simulink library "Lib_PFSys_GenericGenerator_NoSolver"  (R2019b)
settings: Solver=ode45  StartTime=0.0  StopTime=10.0  RelTol=1e-3  EnableMultiTasking=on
Description:
  | Thomas Modules
settings Model: Creator=jwchapm2  LastModifiedBy=mebell
settings DataIOCC: LimitDataPoints=on  SaveFormat=Array  ReturnWorkspaceOutputs=off
settings OptimizationCC: ExpressionDepthLimit=2147483647  LifeSpan=inf
settings DebuggingCC: UnderspecifiedInitializationDetection=Classic  MergeDetectMultiDrivingBlocksExec=none  SolverPrmCheckMsg=warning  StateNameClashWarn=warning  SFUnexpectedBacktrackingDiag=warning  SFNoUnconditionalDefaultTransitionDiag=warning  SFExecutionAtInitializationDiag=none  ArithmeticOperatorsInVariantConditions=warning
settings HardwareCC: ProdBitPerPointer=32  ProdBitPerSizeT=32  ProdBitPerPtrDiffT=32  ProdLargestAtomicFloat=None  ProdIntDivRoundTo=Undefined  ProdEndianess=Unspecified  ProdWordSize=32  ProdHWDeviceType=32-bit Generic
settings ModelReferenceCC: PropagateSignalLabelsOutOfModel=off
settings SFSimCC: SimUseLocalCustomCode=off  CustomCodeUndefinedFunction=UseInterfaceOnly
settings RTWCC: RTWUseLocalCustomCode=off
settings CodeAppCC: StateflowObjectComments=on
settings GRTTargetCC: TargetLangStandard=C89/C90 (ANSI)  GeneratePreprocessorConditionals=Disable all
settings ConfigComp: CovMetricSettings=dw  CovHtmlReporting=on  CovSaveCumulativeToWorkspaceVar=on  CovSaveSingleToWorkspaceVar=on  CovExternalEMLEnable=off

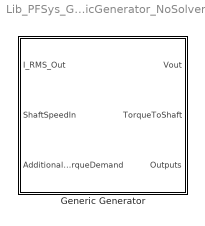
== system Lib_PFSys_GenericGenerator_NoSolver ==
  Generic Generator : Subsystem  mask(Motor){X_C_SpeedVec_M=[0.0 0.1 1.0], Y_C_TorqueVec_M=[0.0 0.1 1.0], T_C_EffArray_M=[0.5 0.5 0.5; 0.5 1.0 1.0; 0.5 1.0 1.0], Ke_M=0.5}
      mask prompts: X_C_SpeedVec_M "X_C_SpeedVec_M - Efficiency Table Speed Vector (X-axis)(nx1)"; Y_C_TorqueVec_M "Y_C_TorqueVec_M - Efficiency Table Torque Vector (Y-axis)(mx1)"; T_C_EffArray_M "T_C_EffArray_M - Efficiency Table Values (Eff = f(i, V)(nxm)"; Ke_M "Ke_M - Motor EMF Constant (V/ rad/s)"
      mask help:
      | This block represents a generic motor with a purely resistive input
      | impedance, and a lumped efficiency/loss model, specified as a lookup table.

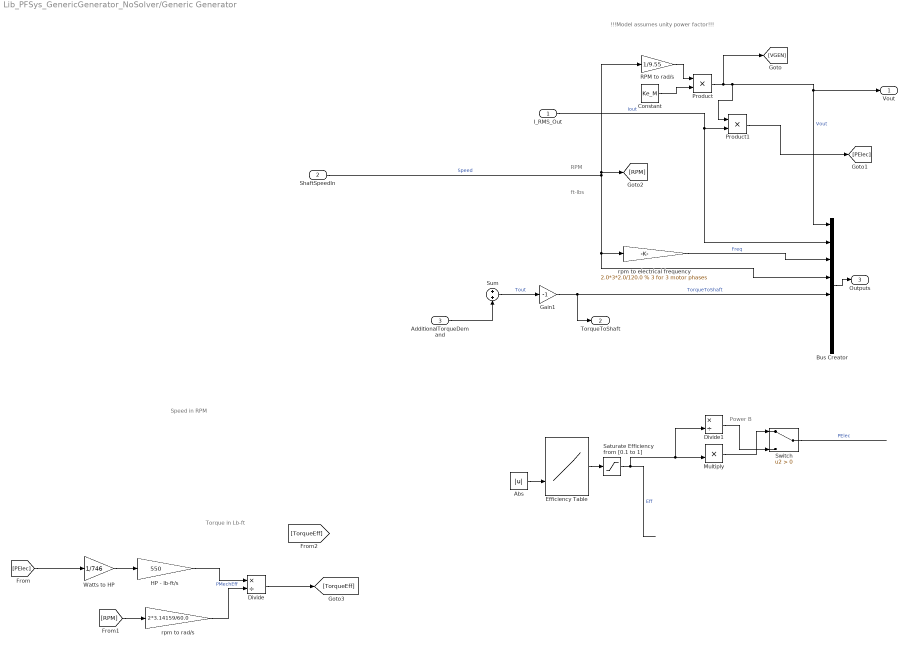
== system Lib_PFSys_GenericGenerator_NoSolver/Generic Generator ==
  note: ft-lbs
  note: RPM
  note: !!!Model assumes unity power factor!!!
  note: Speed in RPM
  note: Torque in Lb-ft
  note: Power B
  I_RMS_Out : Inport
  ShaftSpeedIn : Inport  Port=2
  AdditionalTorqueDemand : Inport  Port=3
  Abs : Abs
  Bus Creator : BusCreator  Inputs=8
  Constant : Constant  Value=Ke_M
  Divide : Product  Inputs=*/
  Divide1 : Product  Inputs=*/
  Efficiency Table : Lookup_n-D  BreakpointsForDimension1=X_C_SpeedVec_M  BreakpointsForDimension2=Y_C_TorqueVec_M  Table=T_C_EffArray_M  ExtrapMethod=Clip  InternalRulePriority=Speed  RndMeth=Simplest  InputSameDT=on
  Gain1 : Gain  Gain=-1
  HP - lb-ft/s : Gain  Gain=550
  Multiply : Product
  Product : Product
  Product1 : Product
  RPM to rad/s : Gain  Gain=1/9.55
  Saturate Efficiency from [0.1 to 1] : Saturate  UpperLimit=1  LowerLimit=0.1
  Sum : Sum
  Switch : Switch  Criteria=u2 > Threshold
  Watts to HP : Gain  Gain=1/746
  rpm to electrical frequency : Gain  Gain=2.0*3*2.0/120.0 % 3 for 3 motor phases
  rpm to rad/s : Gain  Gain=2*3.14159/60.0
  Vout : Outport
  TorqueToShaft : Outport  Port=2
  Outputs : Outport  Port=3  VectorParamsAs1DForOutWhenUnconnected=off
  wires:
  ? -> Bus Creator/7  "PElec"
  Bus Creator/1 -> Outputs/1
  rpm to electrical frequency/1 -> Bus Creator/3  "Freq"
  ShaftSpeedIn/1 -> [RPM], RPM to rad/s/1, Bus Creator/4, rpm to electrical frequency/1  "Speed"
  Product/1 -> Product1/1, Vout/1, Bus Creator/1, [VGEN]  "Vout"
  ? -> Bus Creator/6  "Eff"
  ? -> Bus Creator/8  "PMech"
  RPM to rad/s/1 -> Product/1
  Constant/1 -> Product/2
  Gain1/1 -> Bus Creator/5, TorqueToShaft/1  "TorqueToShaft"
  I_RMS_Out/1 -> Product1/2, Bus Creator/2  "Iout"
  AdditionalTorqueDemand/1 -> Sum/2
  Sum/1 -> Gain1/1  "Tout"
  Product1/1 -> [PElec]
  Multiply/1 -> Switch/1
  ? -> Switch/2, Multiply/1, Divide1/1
  Divide1/1 -> Switch/3
  Saturate Efficiency from [0.1 to 1]/1 -> Divide1/2, Multiply/2  "Eff"
  ? -> Abs/1
  Switch/1 -> ?  "PElec"
  Efficiency Table/1 -> Saturate Efficiency from [0.1 to 1]/1
  Abs/1 -> Efficiency Table/2
  ? -> Efficiency Table/1
  [RPM] -> rpm to rad/s/1
  HP - lb-ft/s/1 -> Divide/1  "PMechEff"
  Watts to HP/1 -> HP - lb-ft/s/1
  [PElec] -> Watts to HP/1
  rpm to rad/s/1 -> Divide/2
  Divide/1 -> [TorqueEff]
